simulink model "decimation_filter_o"  (R2019b)
settings: Solver=VariableStepAuto  StartTime=0.0  StopTime=ts*N*(Mpoints/N+200)  RelTol=1e-3
InitFcn:
  | %fs=256*2e4;
  | %osr=512;
  | 
  | osr=1500;
  | fs=6e6;
  | ts=1/fs;
  | 
  | Ncycle=11;
  | Mpoints=2^15;
  | fin=fs*Ncycle/Mpoints;
  | 
  | N=1024;
  | 
  | ref=16/15;
undefined symbols (not defined in the file or in its folder): argo, clock, firhalfband
libraries: SDtoolbox x19, dspfdesign x9, dspmlti4 x9
settings Model: Creator=admin  LastModifiedBy=admin

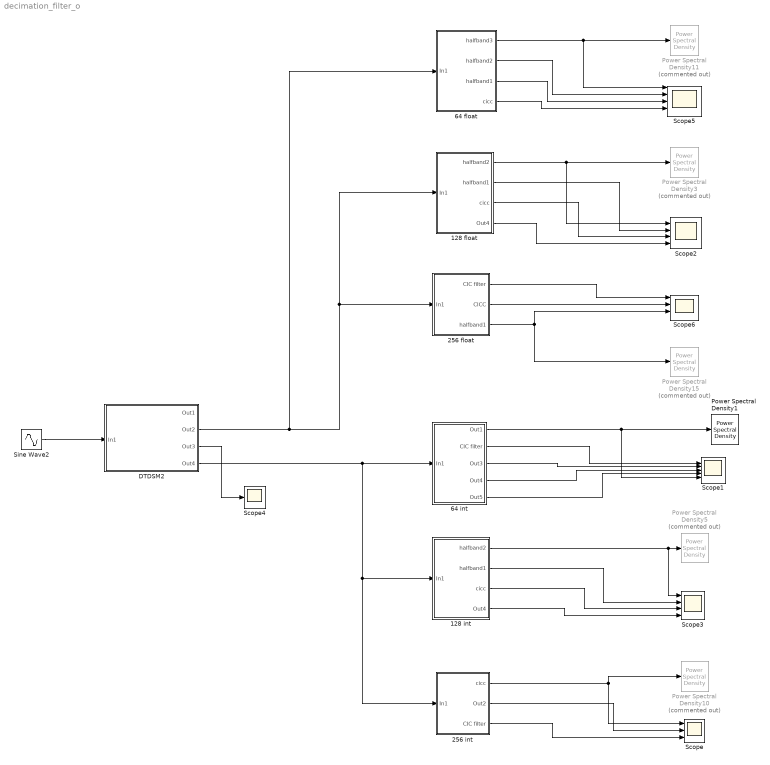
== system decimation_filter_o ==
  "128 float " : Subsystem
  128 int : Subsystem
  256 float : Subsystem
  256 int : Subsystem
  64 float : Subsystem
  64 int : Subsystem
  DTDSM2 : Subsystem
  Power Spectral Density1 : SDtoolbox/Power Spectral Density  SN=7  Fs=fs/1024  fBL=1  fBH=fs/2048  Fin=fin  N=Mpoints/1024  Ntransient=100  VW=on  savename=11  Scale_type=logarithmic
      settings: SourceProductName=SDtoolbox
  Power Spectral Density10 : SDtoolbox/Power Spectral Density  Commented=on  SN=8  Fs=fs/1024  fBL=1  fBH=fs/2048  Fin=fin  N=Mpoints/1024  Ntransient=100  VW=on  savename=11  Scale_type=logarithmic
      settings: SourceProductName=SDtoolbox
  Power Spectral Density11 : SDtoolbox/Power Spectral Density  Commented=on  SN=9  Fs=fs/1024  fBL=1  fBH=fs/2048  Fin=fin  N=Mpoints/1024  Ntransient=100  VW=on  savename=11  Scale_type=logarithmic
      settings: SourceProductName=SDtoolbox
  Power Spectral Density15 : SDtoolbox/Power Spectral Density  Commented=on  SN=10  Fs=fs/1024  fBL=1  fBH=fs/2048  Fin=fin  N=Mpoints/1024  Ntransient=100  VW=on  savename=11  Scale_type=logarithmic
      settings: SourceProductName=SDtoolbox
  Power Spectral Density3 : SDtoolbox/Power Spectral Density  Commented=on  SN=6  Fs=fs/1024  fBL=1  fBH=fs/2048  Fin=fin  N=Mpoints/1024  Ntransient=100  VW=on  savename=11  Scale_type=logarithmic
      settings: SourceProductName=SDtoolbox
  Power Spectral Density5 : SDtoolbox/Power Spectral Density  Commented=on  SN=7  Fs=fs/1024  fBL=1  fBH=fs/2048  Fin=fin  N=Mpoints/1024  Ntransient=100  VW=on  savename=11  Scale_type=logarithmic
      settings: SourceProductName=SDtoolbox
  Scope : Scope  NumInputPorts=3
  Scope1 : Scope  NumInputPorts=5
  Scope2 : Scope  NumInputPorts=4
  Scope3 : Scope  NumInputPorts=4
  Scope4 : Scope
  Scope5 : Scope  NumInputPorts=5
  Scope6 : Scope  NumInputPorts=4
  Sine Wave2 : Sin  Amplitude=0.68  Frequency=fin*2*pi  SampleTime=ts
  wires:
  Sine Wave2/1 -> DTDSM2/1(In1)
  DTDSM2/2(Out2) -> 256 float/1(In1), "128 float "/1(In1), 64 float/1(In1)
  DTDSM2/4(Out4) -> 128 int/1(In1), 256 int/1(In1), 64 int/1(In1)
  "128 float "/1(halfband2) -> Power Spectral Density3/1, Scope2/1
  "128 float "/2(halfband1) -> Scope2/2
  "128 float "/3(cicc) -> Scope2/3
  "128 float "/4(Out4) -> Scope2/4
  128 int/1(halfband2) -> Scope3/1, Power Spectral Density5/1
  128 int/2(halfband1) -> Scope3/2
  128 int/3(cicc) -> Scope3/3
  128 int/4(Out4) -> Scope3/4
  64 float/1(halfband3) -> Power Spectral Density11/1, Scope5/1
  64 float/2(halfband2) -> Scope5/2
  64 float/3(halfband1) -> Scope5/3
  64 float/4(cicc) -> Scope5/4
  256 float/3(halfband1) -> Power Spectral Density15/1, Scope6/3
  256 float/1(CIC filter) -> Scope6/1
  256 float/2(CICC) -> Scope6/2
  256 int/1(cicc) -> Power Spectral Density10/1, Scope/1
  256 int/2(Out2) -> Scope/2
  256 int/3(CIC filter) -> Scope/3
  64 int/2(CIC filter) -> Scope1/1
  64 int/3(Out3) -> Scope1/2
  64 int/4(Out4) -> Scope1/3
  64 int/5(Out5) -> Scope1/4
  DTDSM2/3(Out3) -> Scope4/1
  64 int/1(Out1) -> Power Spectral Density1/1, Scope1/5

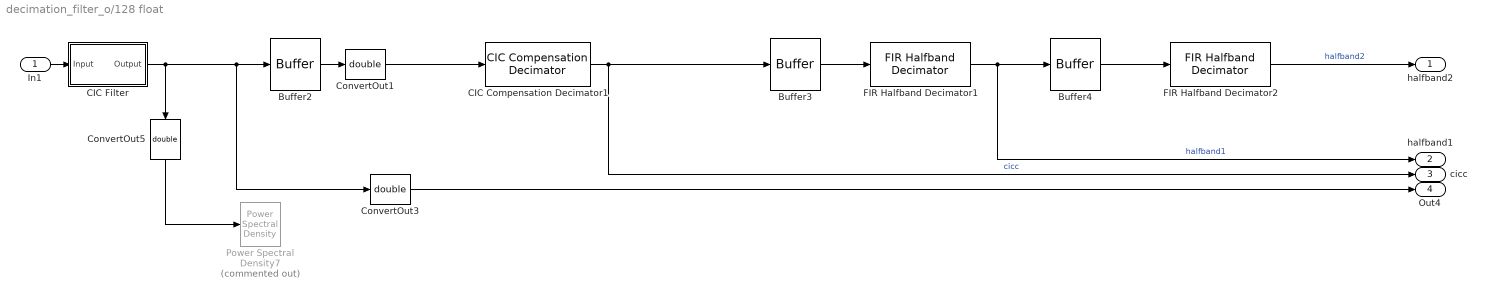
== system decimation_filter_o/128 float  ==
  In1 : Inport
  Buffer2 : Buffer  N=2  OutputFrames=off
  Buffer3 : Buffer  N=2  OutputFrames=off
  Buffer4 : Buffer  N=2  OutputFrames=off
  CIC Compensation Decimator1 : dspfdesign/CIC Compensation Decimator  CICRateChangeFactor=128  CICNumSections=3  CICDifferentialDelay=1  DecimationFactor=2  DesignForMinimumOrder=on  FilterOrder=12  PassbandFrequency=fs/2048  StopbandFrequency=20000  PassbandRipple=0.01  StopbandAttenuation=120  InheritSampleRate=off  SampleRate=23437.5*2  SimulateUsing=Code generation  roundingMode=Floor  coeffsDataTypeStr=fixdt(1,16)
      settings: SourceProductName=DSP System Toolbox  SourceProductBaseCode=DS
  CIC Filter : Subsystem  Tag=FilterWizardSubSystem
      settings: ErrorFcn=dspFilterRealizedInBasicElemsAlgLoopErrFcnCallback
  ConvertOut1 : DataTypeConversion  OutDataTypeStr=double
  ConvertOut3 : DataTypeConversion  OutDataTypeStr=double
  ConvertOut5 : DataTypeConversion  OutDataTypeStr=double
  FIR Halfband Decimator1 : dspfdesign/FIR Halfband Decimator  Specification=Transition width and stopband attenuation  FilterOrder=52  TransitionWidth=6000  StopbandAttenuation=80  Numerator=firhalfband( 'minorder', 0.407, 1e-4 )  FilterBankOutputPort=off  InheritSampleRate=off  SampleRate=fs/256  SimulateUsing=Code generation  roundingMode=Floor  coeffsDataTypeStr=fixdt(1,16)
      settings: SourceProductName=DSP System Toolbox  SourceProductBaseCode=DS
  FIR Halfband Decimator2 : dspfdesign/FIR Halfband Decimator  Specification=Transition width and stopband attenuation  FilterOrder=52  TransitionWidth=3000  StopbandAttenuation=90  Numerator=firhalfband( 'minorder', 0.407, 1e-4 )  FilterBankOutputPort=off  InheritSampleRate=off  SampleRate=fs/512  SimulateUsing=Code generation  roundingMode=Floor  coeffsDataTypeStr=fixdt(1,16)
      settings: SourceProductName=DSP System Toolbox  SourceProductBaseCode=DS
  Power Spectral Density7 : SDtoolbox/Power Spectral Density  Commented=on  SN=5  Fs=fs/128  fBL=1  fBH=fs/2048  Fin=fin  N=Mpoints/128  Ntransient=100  VW=on  savename=11  Scale_type=logarithmic
      settings: SourceProductName=SDtoolbox
  halfband2 : Outport
  halfband1 : Outport  Port=2
  cicc : Outport  Port=3
  Out4 : Outport  Port=4
  wires:
  ConvertOut1/1 -> CIC Compensation Decimator1/1
  Buffer3/1 -> FIR Halfband Decimator1/1
  CIC Filter/1(Output) -> ConvertOut5/1, Buffer2/1, ConvertOut3/1
  FIR Halfband Decimator2/1 -> halfband2/1  "halfband2"
  FIR Halfband Decimator1/1 -> halfband1/1, Buffer4/1  "halfband1"
  ConvertOut5/1 -> Power Spectral Density7/1
  Buffer2/1 -> ConvertOut1/1
  Buffer4/1 -> FIR Halfband Decimator2/1
  CIC Compensation Decimator1/1 -> cicc/1, Buffer3/1  "cicc"
  ConvertOut3/1 -> Out4/1
  In1/1 -> CIC Filter/1(Input)

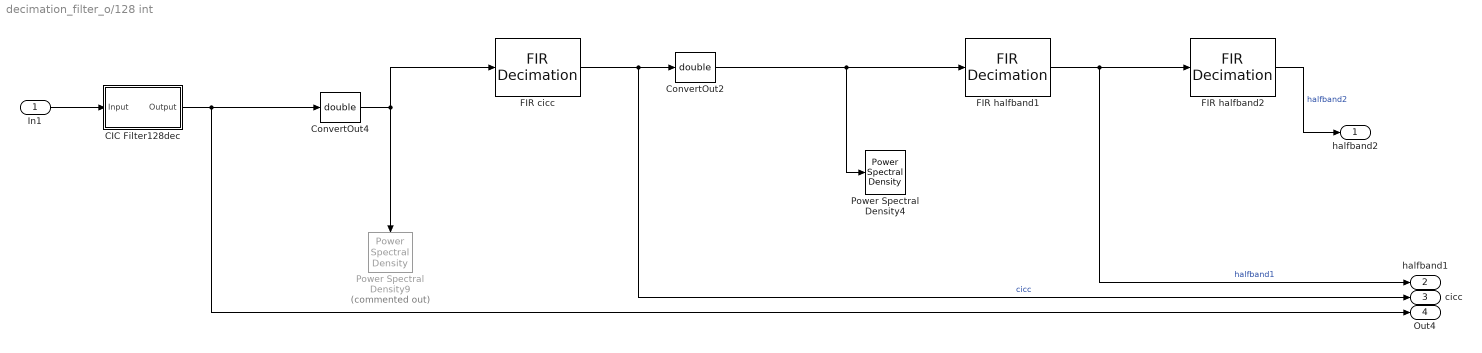
== system decimation_filter_o/128 int ==
  In1 : Inport
  CIC Filter128dec : Subsystem  Tag=FilterWizardSubSystem
      settings: ErrorFcn=dspFilterRealizedInBasicElemsAlgLoopErrFcnCallback
  ConvertOut2 : DataTypeConversion  OutDataTypeStr=double
  ConvertOut4 : DataTypeConversion  OutDataTypeStr=double
  FIR cicc : dspmlti4/FIR Decimation  FilterSource=Dialog parameters  h=coff_ciccom_round_128m  D=2  filtStruct=Direct form  FilterObject=FDECIM  framing=Allow multirate processing  inputOffset=0  outputBufInitCond=0  roundingMode=Ceiling  overflowMode=off  firstCoeffDataTypeStr=Inherit: Same word length as input  firstCoeffMin=[]  firstCoeffMax=[]  firstCoeffLastDataTypeStr=Inherit: Same word length as input  outputMin=[]  outputMax=[]
  FIR halfband1 : dspmlti4/FIR Decimation  FilterSource=Dialog parameters  h=half1co_r_128m  D=2  filtStruct=Direct form  FilterObject=FDECIM  framing=Allow multirate processing  inputOffset=0  outputBufInitCond=0  roundingMode=Ceiling  overflowMode=off  firstCoeffDataTypeStr=Inherit: Same word length as input  firstCoeffMin=[]  firstCoeffMax=[]  firstCoeffLastDataTypeStr=Inherit: Same word length as input  outputMin=[]  outputMax=[]
  FIR halfband2 : dspmlti4/FIR Decimation  FilterSource=Dialog parameters  h=half2co_r_128m  D=2  filtStruct=Direct form  FilterObject=FDECIM  framing=Allow multirate processing  inputOffset=0  outputBufInitCond=0  roundingMode=Ceiling  overflowMode=off  firstCoeffDataTypeStr=Inherit: Same word length as input  firstCoeffMin=[]  firstCoeffMax=[]  firstCoeffLastDataTypeStr=Inherit: Same word length as input  outputMin=[]  outputMax=[]
  Power Spectral Density4 : SDtoolbox/Power Spectral Density  SN=5  Fs=fs/256  fBL=1  fBH=fs/2048  Fin=fin  N=Mpoints/256  Ntransient=100  VW=on  savename=11  Scale_type=logarithmic
      settings: SourceProductName=SDtoolbox
  Power Spectral Density9 : SDtoolbox/Power Spectral Density  Commented=on  SN=5  Fs=fs/128  fBL=1  fBH=fs/2048  Fin=fin  N=Mpoints/128  Ntransient=100  VW=on  savename=11  Scale_type=logarithmic
      settings: SourceProductName=SDtoolbox
  halfband2 : Outport
  halfband1 : Outport  Port=2
  cicc : Outport  Port=3
  Out4 : Outport  Port=4
  wires:
  In1/1 -> CIC Filter128dec/1(Input)
  FIR halfband1/1 -> halfband1/1, FIR halfband2/1  "halfband1"
  FIR cicc/1 -> cicc/1, ConvertOut2/1  "cicc"
  ConvertOut4/1 -> Power Spectral Density9/1, FIR cicc/1
  FIR halfband2/1 -> halfband2/1  "halfband2"
  CIC Filter128dec/1(Output) -> Out4/1, ConvertOut4/1
  ConvertOut2/1 -> Power Spectral Density4/1, FIR halfband1/1

== system decimation_filter_o/256 float ==
  In1 : Inport
  Buffer10 : Buffer  N=2  OutputFrames=off
  Buffer9 : Buffer  N=2  OutputFrames=off
  CIC Compensation Decimator3 : dspfdesign/CIC Compensation Decimator  CICRateChangeFactor=256  CICNumSections=3  CICDifferentialDelay=1  DecimationFactor=2  DesignForMinimumOrder=on  FilterOrder=12  PassbandFrequency=fs/2048  StopbandFrequency=10000  PassbandRipple=0.01  StopbandAttenuation=120  InheritSampleRate=off  SampleRate=23437.5  SimulateUsing=Code generation  roundingMode=Floor  coeffsDataTypeStr=fixdt(1,16)
      settings: SourceProductName=DSP System Toolbox  SourceProductBaseCode=DS
  ConvertOut9 : DataTypeConversion  OutDataTypeStr=double
  FIR Halfband Decimator6 : dspfdesign/FIR Halfband Decimator  Specification=Transition width and stopband attenuation  FilterOrder=52  TransitionWidth=4000  StopbandAttenuation=90  Numerator=firhalfband( 'minorder', 0.407, 1e-4 )  FilterBankOutputPort=off  InheritSampleRate=off  SampleRate=fs/512  SimulateUsing=Code generation  roundingMode=Floor  coeffsDataTypeStr=fixdt(1,16)
      settings: SourceProductName=DSP System Toolbox  SourceProductBaseCode=DS
  Filter1 : Subsystem  Tag=FilterWizardSubSystem
      settings: ErrorFcn=dspFilterRealizedInBasicElemsAlgLoopErrFcnCallback
  Power Spectral Density12 : SDtoolbox/Power Spectral Density  Commented=on  SN=3  Fs=fs/256  fBL=1  fBH=fs/2048  Fin=fin  N=Mpoints/256  Ntransient=10  VW=on  savename=11  Scale_type=logarithmic
      settings: SourceProductName=SDtoolbox
  Power Spectral Density13 : SDtoolbox/Power Spectral Density  Commented=on  SN=4  Fs=fs/512  fBL=1  fBH=fs/2048  Fin=fin  N=Mpoints/512  Ntransient=10  VW=on  savename=11  Scale_type=logarithmic
      settings: SourceProductName=SDtoolbox
  CIC filter : Outport
  CICC : Outport  Port=2
  halfband1 : Outport  Port=3
  wires:
  ConvertOut9/1 -> Power Spectral Density12/1, CIC Compensation Decimator3/1
  CIC Compensation Decimator3/1 -> CICC/1, Buffer10/1, Power Spectral Density13/1  "CICC"
  Filter1/1(Output) -> CIC filter/1, Buffer9/1  "CIC filter"
  Buffer9/1 -> ConvertOut9/1
  Buffer10/1 -> FIR Halfband Decimator6/1
  In1/1 -> Filter1/1(Input)
  FIR Halfband Decimator6/1 -> halfband1/1  "halfband1"

== system decimation_filter_o/256 int ==
  In1 : Inport
  CIC Filter256dec : Subsystem  Tag=FilterWizardSubSystem
      settings: ErrorFcn=dspFilterRealizedInBasicElemsAlgLoopErrFcnCallback
  ConvertOut6 : DataTypeConversion  OutDataTypeStr=double
  FIR cicc1 : dspmlti4/FIR Decimation  FilterSource=Dialog parameters  h=coff_ciccom_round_256m  D=2  filtStruct=Direct form  FilterObject=FDECIM  framing=Allow multirate processing  inputOffset=0  outputBufInitCond=0  roundingMode=Ceiling  overflowMode=off  firstCoeffDataTypeStr=Inherit: Same word length as input  firstCoeffMin=[]  firstCoeffMax=[]  firstCoeffLastDataTypeStr=Inherit: Same word length as input  outputMin=[]  outputMax=[]
  FIR halfband : dspmlti4/FIR Decimation  FilterSource=Dialog parameters  h=half1co_r_256m  D=2  filtStruct=Direct form  FilterObject=FDECIM  framing=Allow multirate processing  inputOffset=0  outputBufInitCond=0  roundingMode=Ceiling  overflowMode=off  firstCoeffDataTypeStr=Inherit: Same word length as input  firstCoeffMin=[]  firstCoeffMax=[]  firstCoeffLastDataTypeStr=Inherit: Same word length as input  outputMin=[]  outputMax=[]
  Power Spectral Density6 : SDtoolbox/Power Spectral Density  Commented=on  SN=5  Fs=fs/256  fBL=1  fBH=fs/2048  Fin=fin  N=Mpoints/256  Ntransient=100  VW=on  savename=11  Scale_type=logarithmic
      settings: SourceProductName=SDtoolbox
  cicc : Outport
  Out2 : Outport  Port=2
  CIC filter : Outport  Port=3
  wires:
  ConvertOut6/1 -> Power Spectral Density6/1, FIR cicc1/1
  FIR cicc1/1 -> Out2/1, FIR halfband/1
  In1/1 -> CIC Filter256dec/1(Input)
  CIC Filter256dec/1(Output) -> CIC filter/1, ConvertOut6/1  "CIC filter"
  FIR halfband/1 -> cicc/1  "cicc"

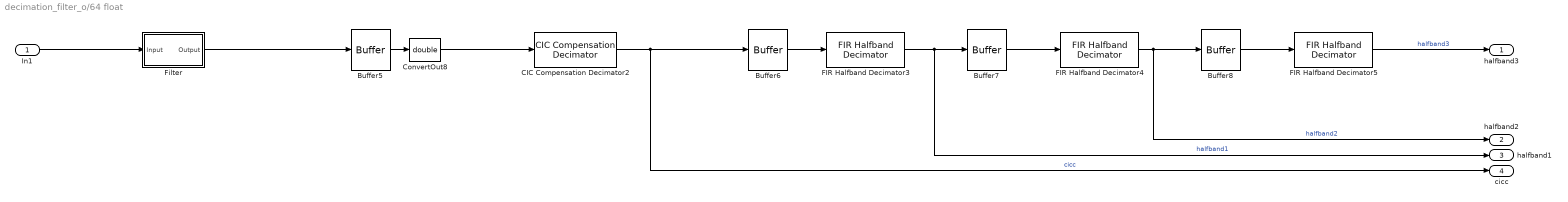
== system decimation_filter_o/64 float ==
  In1 : Inport
  Buffer{5..8} (4 alike) : Buffer  N=2  OutputFrames=off
  CIC Compensation Decimator2 : dspfdesign/CIC Compensation Decimator  CICRateChangeFactor=64  CICNumSections=3  CICDifferentialDelay=1  DecimationFactor=2  DesignForMinimumOrder=on  FilterOrder=12  PassbandFrequency=fs/2048  StopbandFrequency=40000  PassbandRipple=0.01  StopbandAttenuation=120  InheritSampleRate=off  SampleRate=23437.5*4  SimulateUsing=Code generation  roundingMode=Floor  coeffsDataTypeStr=fixdt(1,16)
      settings: SourceProductName=DSP System Toolbox  SourceProductBaseCode=DS
  ConvertOut8 : DataTypeConversion  OutDataTypeStr=double
  FIR Halfband Decimator3 : dspfdesign/FIR Halfband Decimator  Specification=Transition width and stopband attenuation  FilterOrder=52  TransitionWidth=16000  StopbandAttenuation=80  Numerator=firhalfband( 'minorder', 0.407, 1e-4 )  FilterBankOutputPort=off  InheritSampleRate=off  SampleRate=fs/128  SimulateUsing=Code generation  roundingMode=Floor  coeffsDataTypeStr=fixdt(1,16)
      settings: SourceProductName=DSP System Toolbox  SourceProductBaseCode=DS
  FIR Halfband Decimator4 : dspfdesign/FIR Halfband Decimator  Specification=Transition width and stopband attenuation  FilterOrder=52  TransitionWidth=10000  StopbandAttenuation=90  Numerator=firhalfband( 'minorder', 0.407, 1e-4 )  FilterBankOutputPort=off  InheritSampleRate=off  SampleRate=fs/256  SimulateUsing=Code generation  roundingMode=Floor  coeffsDataTypeStr=fixdt(1,16)
      settings: SourceProductName=DSP System Toolbox  SourceProductBaseCode=DS
  FIR Halfband Decimator5 : dspfdesign/FIR Halfband Decimator  Specification=Transition width and stopband attenuation  FilterOrder=52  TransitionWidth=3500  StopbandAttenuation=100  Numerator=firhalfband( 'minorder', 0.407, 1e-4 )  FilterBankOutputPort=off  InheritSampleRate=off  SampleRate=fs/512  SimulateUsing=Code generation  roundingMode=Floor  coeffsDataTypeStr=fixdt(1,16)
      settings: SourceProductName=DSP System Toolbox  SourceProductBaseCode=DS
  Filter : Subsystem  Tag=FilterWizardSubSystem
      settings: ErrorFcn=dspFilterRealizedInBasicElemsAlgLoopErrFcnCallback
  halfband3 : Outport
  halfband2 : Outport  Port=2
  halfband1 : Outport  Port=3
  cicc : Outport  Port=4
  wires:
  Buffer8/1 -> FIR Halfband Decimator5/1
  Buffer7/1 -> FIR Halfband Decimator4/1
  FIR Halfband Decimator4/1 -> halfband2/1, Buffer8/1  "halfband2"
  Filter/1(Output) -> Buffer5/1
  CIC Compensation Decimator2/1 -> cicc/1, Buffer6/1  "cicc"
  FIR Halfband Decimator3/1 -> halfband1/1, Buffer7/1  "halfband1"
  Buffer6/1 -> FIR Halfband Decimator3/1
  Buffer5/1 -> ConvertOut8/1
  ConvertOut8/1 -> CIC Compensation Decimator2/1
  FIR Halfband Decimator5/1 -> halfband3/1  "halfband3"
  In1/1 -> Filter/1(Input)

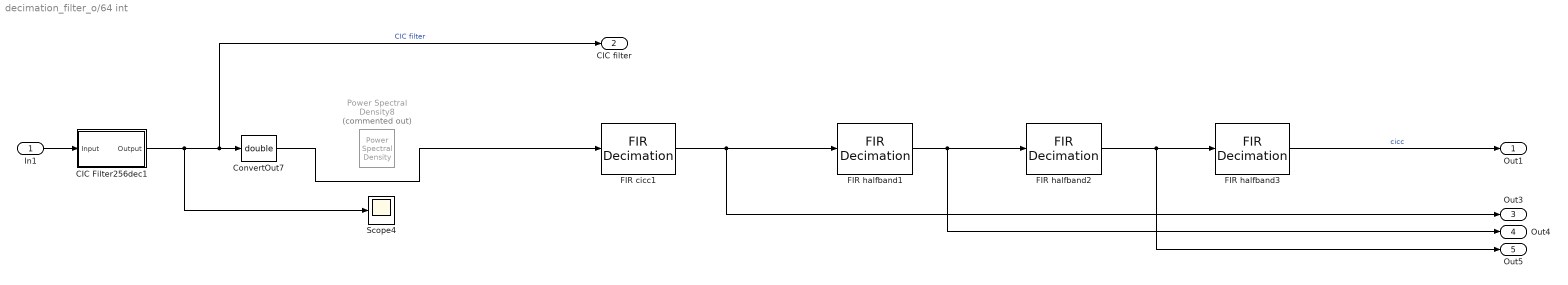
== system decimation_filter_o/64 int ==
  In1 : Inport
  CIC Filter256dec1 : Subsystem  Tag=FilterWizardSubSystem
      settings: ErrorFcn=dspFilterRealizedInBasicElemsAlgLoopErrFcnCallback
  ConvertOut7 : DataTypeConversion  OutDataTypeStr=double
  FIR cicc1 : dspmlti4/FIR Decimation  FilterSource=Dialog parameters  h=coff_ciccom_round_64m  D=2  filtStruct=Direct form  FilterObject=FDECIM  framing=Allow multirate processing  inputOffset=0  outputBufInitCond=0  roundingMode=Ceiling  overflowMode=off  firstCoeffDataTypeStr=Inherit: Same word length as input  firstCoeffMin=[]  firstCoeffMax=[]  firstCoeffLastDataTypeStr=Inherit: Same word length as input  outputMin=[]  outputMax=[]
  FIR halfband1 : dspmlti4/FIR Decimation  FilterSource=Dialog parameters  h=half1co_r_64m  D=2  filtStruct=Direct form  FilterObject=FDECIM  framing=Allow multirate processing  inputOffset=0  outputBufInitCond=0  roundingMode=Ceiling  overflowMode=off  firstCoeffDataTypeStr=Inherit: Same word length as input  firstCoeffMin=[]  firstCoeffMax=[]  firstCoeffLastDataTypeStr=Inherit: Same word length as input  outputMin=[]  outputMax=[]
  FIR halfband2 : dspmlti4/FIR Decimation  FilterSource=Dialog parameters  h=half2co_r_64m  D=2  filtStruct=Direct form  FilterObject=FDECIM  framing=Allow multirate processing  inputOffset=0  outputBufInitCond=0  roundingMode=Ceiling  overflowMode=off  firstCoeffDataTypeStr=Inherit: Same word length as input  firstCoeffMin=[]  firstCoeffMax=[]  firstCoeffLastDataTypeStr=Inherit: Same word length as input  outputMin=[]  outputMax=[]
  FIR halfband3 : dspmlti4/FIR Decimation  FilterSource=Dialog parameters  h=half3co_r_64m  D=2  filtStruct=Direct form  FilterObject=FDECIM  framing=Allow multirate processing  inputOffset=0  outputBufInitCond=0  roundingMode=Ceiling  overflowMode=off  firstCoeffDataTypeStr=Inherit: Same word length as input  firstCoeffMin=[]  firstCoeffMax=[]  firstCoeffLastDataTypeStr=Inherit: Same word length as input  outputMin=[]  outputMax=[]
  Power Spectral Density8 : SDtoolbox/Power Spectral Density  Commented=on  SN=5  Fs=fs/64  fBL=1  fBH=fs/2048  Fin=fin  N=Mpoints/64  Ntransient=100  VW=on  savename=11  Scale_type=logarithmic
      settings: SourceProductName=SDtoolbox
  Scope4 : Scope
  Out1 : Outport
  CIC filter : Outport  Port=2
  Out3 : Outport  Port=3
  Out4 : Outport  Port=4
  Out5 : Outport  Port=5
  wires:
  FIR cicc1/1 -> Out3/1, FIR halfband1/1
  FIR halfband3/1 -> Out1/1  "cicc"
  FIR halfband2/1 -> Out5/1, FIR halfband3/1
  CIC Filter256dec1/1(Output) -> Scope4/1, CIC filter/1, ConvertOut7/1  "CIC filter"
  FIR halfband1/1 -> Out4/1, FIR halfband2/1
  In1/1 -> CIC Filter256dec1/1(Input)
  ConvertOut7/1 -> FIR cicc1/1

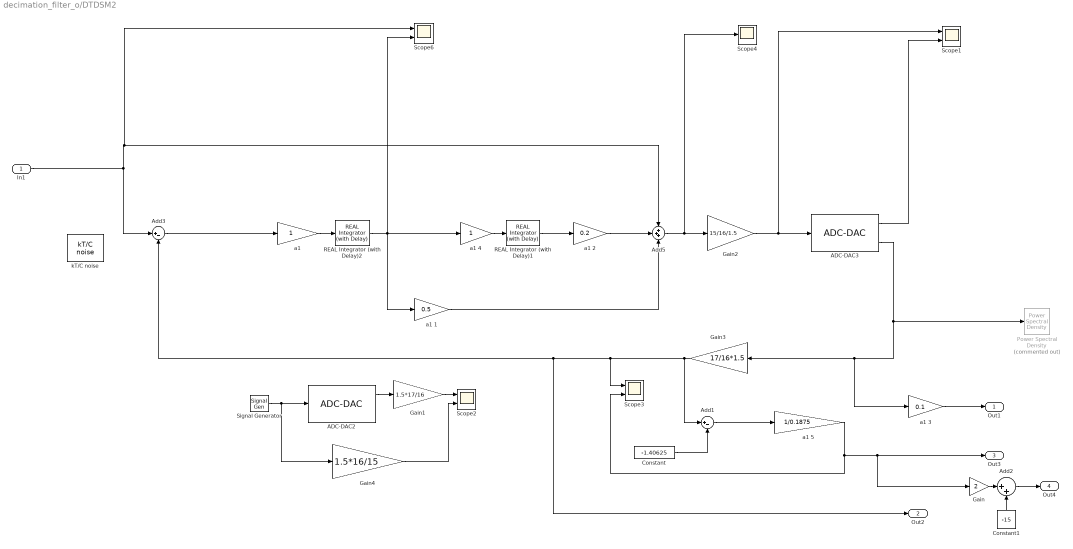
== system decimation_filter_o/DTDSM2 ==
  In1 : Inport
  ADC-DAC2 : SDtoolbox/ADC-DAC  k=17  MM=off  match=0  CST=0  VVG=off  argo=argo(:,3)  LF=on  NF=retA.log
      settings: SourceProductName=SDtoolbox
  ADC-DAC3 : SDtoolbox/ADC-DAC  k=17  MM=off  match=0  CST=0  VVG=off  argo=argo(:,3)  LF=on  NF=retA.log
      settings: SourceProductName=SDtoolbox
  Add1 : Sum  Inputs=|+-
  Add2 : Sum  Inputs=|++
  Add3 : Sum  Inputs=|+-
  Add5 : Sum  Inputs=+++
  Constant : Constant  Value=-1.40625
  Constant1 : Constant  Value=-15
  Gain : Gain  Gain=2
  Gain1 : Gain  Gain=1.5*17/16
  Gain2 : Gain  Gain=15/16/1.5
  Gain3 : Gain  Gain=17/16*1.5
  Gain4 : Gain  Gain=1.5*16/15
  Power Spectral Density : SDtoolbox/Power Spectral Density  Commented=on  SN=3  Fs=fs  fBL=1  fBH=fs/2048  Fin=fin  N=Mpoints  Ntransient=10  VW=on  savename=11  Scale_type=logarithmic
      settings: SourceProductName=SDtoolbox
  REAL Integrator (with Delay)1 : SDtoolbox/REAL Integrator (with Delay)  Ts=ts  alfa=(1e4-1)/1e4  Amax=1  sr=1e7  GBW=1e8
      settings: SourceProductName=SDtoolbox
  REAL Integrator (with Delay)2 : SDtoolbox/REAL Integrator (with Delay)  Ts=ts  alfa=(1e4-1)/1e4  Amax=3.3  sr=1E8  GBW=1E7
      settings: SourceProductName=SDtoolbox
  Scope{1..3,6} (4 alike) : Scope  NumInputPorts=2
  Scope4 : Scope
  Signal Generator : SignalGenerator  WaveForm=sawtooth  Frequency=5000  Units=rad/sec
  "a1 " : Gain
  a1 1 : Gain  Gain=0.5
  a1 2 : Gain  Gain=0.2
  a1 3 : Gain  Gain=0.1
  a1 4 : Gain
  a1 5 : Gain  Gain=1/0.1875
  kT/C noise : SDtoolbox/kT//C noise  Ts=ts  C=16e-12  Temp=300  k=1.38e-23  seed=floor(sum(clock))
      settings: SourceProductName=SDtoolbox
  Out1 : Outport
  Out2 : Outport  Port=2
  Out3 : Outport  Port=3
  Out4 : Outport  Port=4
  wires:
  Gain2/1 -> ADC-DAC3/1, Scope1/1
  Add3/1 -> "a1 "/1
  REAL Integrator (with Delay)1/1 -> a1 2/1
  Gain1/1 -> Scope2/1
  a1 2/1 -> Add5/2
  a1 4/1 -> REAL Integrator (with Delay)1/1
  In1/1 -> Add3/1, Add5/1, Scope6/1
  "a1 "/1 -> REAL Integrator (with Delay)2/1
  Add5/1 -> Scope4/1, Gain2/1
  Signal Generator/1 -> Gain4/1, ADC-DAC2/1
  ADC-DAC3/1 -> Scope1/2
  REAL Integrator (with Delay)2/1 -> a1 4/1, Scope6/2, a1 1/1
  ADC-DAC2/1 -> Gain1/1
  a1 1/1 -> Add5/3
  Gain4/1 -> Scope2/2
  ADC-DAC3/2 -> Power Spectral Density/1, a1 3/1, Gain3/1
  a1 3/1 -> Out1/1
  Gain3/1 -> Add1/1, Scope3/1, Out2/1, Add3/2
  Constant/1 -> Add1/2
  Add1/1 -> a1 5/1
  a1 5/1 -> Gain/1, Out3/1, Scope3/2
  Constant1/1 -> Add2/2
  Gain/1 -> Add2/1
  Add2/1 -> Out4/1

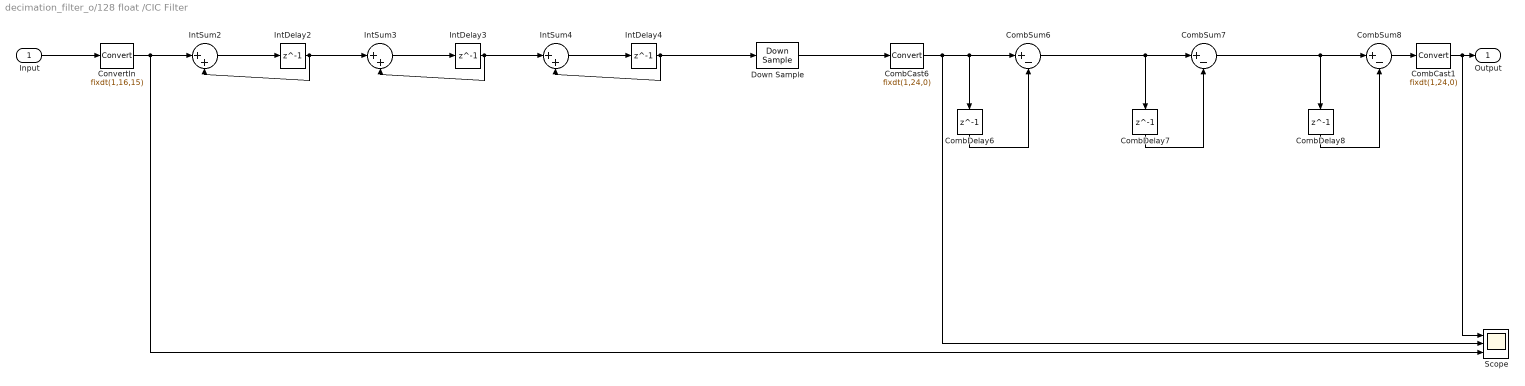
== system decimation_filter_o/128 float /CIC Filter ==
  Input : Inport
  CombCast1 : DataTypeConversion  OutDataTypeStr=fixdt(1,24,0)
  CombCast6 : DataTypeConversion  OutDataTypeStr=fixdt(1,24,0)
  CombDelay6 : Delay  DelayLength=1  InitialCondition=0
  CombDelay7 : Delay  DelayLength=1  InitialCondition=0
  CombDelay8 : Delay  DelayLength=1  InitialCondition=0
  CombSum6 : Sum  Inputs=|+-  AccumDataTypeStr=fixdt(1,37,15)  OutDataTypeStr=fixdt(1,37,15)
  CombSum7 : Sum  Inputs=|+-  AccumDataTypeStr=fixdt(1,37,15)  OutDataTypeStr=fixdt(1,37,15)
  CombSum8 : Sum  Inputs=|+-  AccumDataTypeStr=fixdt(1,37,15)  OutDataTypeStr=fixdt(1,37,15)
  ConvertIn : DataTypeConversion  OutDataTypeStr=fixdt(1,16,15)  RndMeth=Nearest  SaturateOnIntegerOverflow=on
  Down Sample : DownSample  N=128  RateOptions=Allow multirate processing
  IntDelay2 : Delay  DelayLength=1  InitialCondition=0
  IntDelay3 : Delay  DelayLength=1  InitialCondition=0
  IntDelay4 : Delay  DelayLength=1  InitialCondition=0
  IntSum2 : Sum  Inputs=|++  AccumDataTypeStr=fixdt(1,37,15)  OutDataTypeStr=fixdt(1,37,15)
  IntSum3 : Sum  Inputs=|++  AccumDataTypeStr=fixdt(1,37,15)  OutDataTypeStr=fixdt(1,37,15)
  IntSum4 : Sum  Inputs=|++  AccumDataTypeStr=fixdt(1,37,15)  OutDataTypeStr=fixdt(1,37,15)
  Scope : Scope  NumInputPorts=3
  Output : Outport
  wires:
  Input/1 -> ConvertIn/1
  ConvertIn/1 -> Scope/3, IntSum2/1
  IntSum2/1 -> IntDelay2/1
  IntDelay2/1 -> IntSum2/2, IntSum3/1
  IntSum3/1 -> IntDelay3/1
  IntDelay3/1 -> IntSum3/2, IntSum4/1
  IntSum4/1 -> IntDelay4/1
  IntDelay4/1 -> IntSum4/2, Down Sample/1
  Down Sample/1 -> CombCast6/1
  CombSum6/1 -> CombSum7/1, CombDelay7/1
  CombDelay6/1 -> CombSum6/2
  CombCast6/1 -> Scope/2, CombSum6/1, CombDelay6/1
  CombSum7/1 -> CombSum8/1, CombDelay8/1
  CombDelay7/1 -> CombSum7/2
  CombSum8/1 -> CombCast1/1
  CombDelay8/1 -> CombSum8/2
  CombCast1/1 -> Scope/1, Output/1

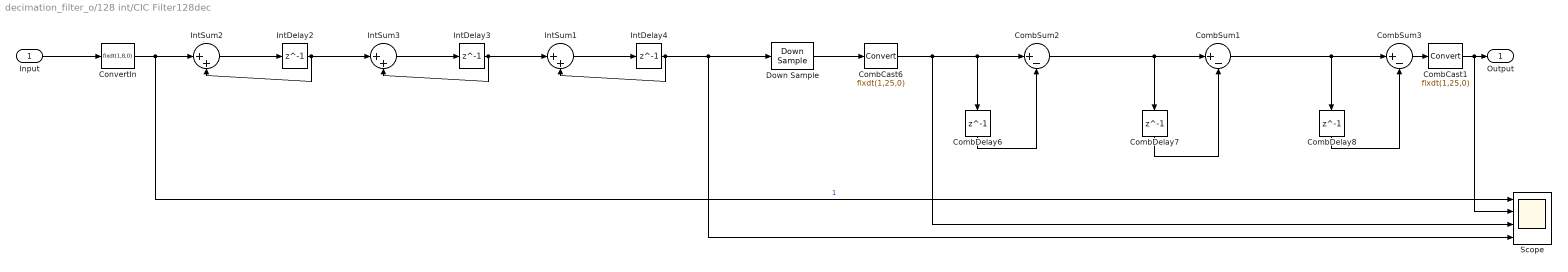
== system decimation_filter_o/128 int/CIC Filter128dec ==
  Input : Inport
  CombCast1 : DataTypeConversion  OutDataTypeStr=fixdt(1,25,0)
  CombCast6 : DataTypeConversion  OutDataTypeStr=fixdt(1,25,0)
  CombDelay6 : Delay  DelayLength=1  InitialCondition=0
  CombDelay7 : Delay  DelayLength=1  InitialCondition=0
  CombDelay8 : Delay  DelayLength=1  InitialCondition=0
  CombSum1 : Sum  Inputs=|+-  AccumDataTypeStr=fixdt(1,25,0)  OutDataTypeStr=fixdt(1,26,0)
  CombSum2 : Sum  Inputs=|+-  AccumDataTypeStr=fixdt(1,25,0)  OutDataTypeStr=fixdt(1,26,0)
  CombSum3 : Sum  Inputs=|+-  AccumDataTypeStr=fixdt(1,25,0)  OutDataTypeStr=fixdt(1,26,0)
  ConvertIn : DataTypeConversion  OutDataTypeStr=fixdt(1,8,0)  RndMeth=Nearest
  Down Sample : DownSample  N=128  RateOptions=Allow multirate processing
  IntDelay2 : Delay  DelayLength=1  InitialCondition=0
  IntDelay3 : Delay  DelayLength=1  InitialCondition=0
  IntDelay4 : Delay  DelayLength=1  InitialCondition=0
  IntSum1 : Sum  Inputs=|++  AccumDataTypeStr=fixdt(1,26,0)  OutDataTypeStr=fixdt(1,26,0)
  IntSum2 : Sum  Inputs=|++  AccumDataTypeStr=fixdt(1,24,0)  OutDataTypeStr=fixdt(1,26,0)
  IntSum3 : Sum  Inputs=|++  AccumDataTypeStr=fixdt(1,26,0)  OutDataTypeStr=fixdt(1,26,0)
  Scope : Scope  NumInputPorts=4
  Output : Outport
  wires:
  ConvertIn/1 -> Scope/1, IntSum2/1  "1"
  IntSum2/1 -> IntDelay2/1
  IntDelay2/1 -> IntSum3/1, IntSum2/2
  IntSum3/1 -> IntDelay3/1
  IntDelay3/1 -> IntSum1/1, IntSum3/2
  IntSum1/1 -> IntDelay4/1
  Down Sample/1 -> CombCast6/1
  CombSum2/1 -> CombSum1/1, CombDelay7/1
  CombDelay6/1 -> CombSum2/2
  CombCast6/1 -> Scope/3, CombSum2/1, CombDelay6/1
  CombSum1/1 -> CombSum3/1, CombDelay8/1
  CombDelay7/1 -> CombSum1/2
  CombSum3/1 -> CombCast1/1
  CombDelay8/1 -> CombSum3/2
  CombCast1/1 -> Scope/2, Output/1
  Input/1 -> ConvertIn/1
  IntDelay4/1 -> IntSum1/2, Scope/4, Down Sample/1

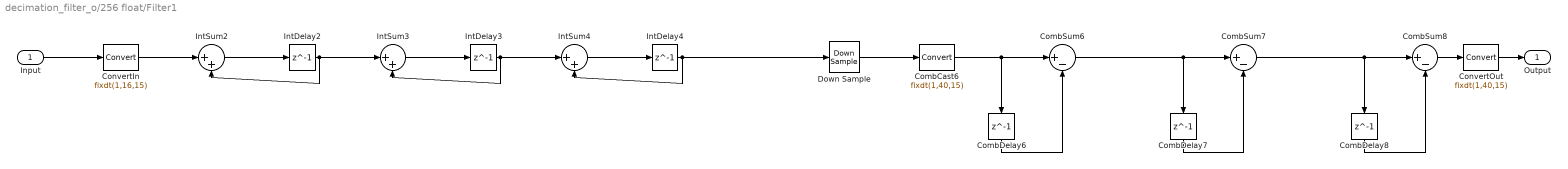
== system decimation_filter_o/256 float/Filter1 ==
  Input : Inport
  CombCast6 : DataTypeConversion  OutDataTypeStr=fixdt(1,40,15)
  CombDelay6 : Delay  DelayLength=1  InitialCondition=0
  CombDelay7 : Delay  DelayLength=1  InitialCondition=0
  CombDelay8 : Delay  DelayLength=1  InitialCondition=0
  CombSum6 : Sum  Inputs=|+-  AccumDataTypeStr=fixdt(1,40,15)  OutDataTypeStr=fixdt(1,40,15)
  CombSum7 : Sum  Inputs=|+-  AccumDataTypeStr=fixdt(1,40,15)  OutDataTypeStr=fixdt(1,40,15)
  CombSum8 : Sum  Inputs=|+-  AccumDataTypeStr=fixdt(1,40,15)  OutDataTypeStr=fixdt(1,40,15)
  ConvertIn : DataTypeConversion  OutDataTypeStr=fixdt(1,16,15)  RndMeth=Nearest  SaturateOnIntegerOverflow=on
  ConvertOut : DataTypeConversion  OutDataTypeStr=fixdt(1,40,15)
  Down Sample : DownSample  N=256  RateOptions=Allow multirate processing
  IntDelay2 : Delay  DelayLength=1  InitialCondition=0
  IntDelay3 : Delay  DelayLength=1  InitialCondition=0
  IntDelay4 : Delay  DelayLength=1  InitialCondition=0
  IntSum2 : Sum  Inputs=|++  AccumDataTypeStr=fixdt(1,40,15)  OutDataTypeStr=fixdt(1,40,15)
  IntSum3 : Sum  Inputs=|++  AccumDataTypeStr=fixdt(1,40,15)  OutDataTypeStr=fixdt(1,40,15)
  IntSum4 : Sum  Inputs=|++  AccumDataTypeStr=fixdt(1,40,15)  OutDataTypeStr=fixdt(1,40,15)
  Output : Outport
  wires:
  Input/1 -> ConvertIn/1
  ConvertIn/1 -> IntSum2/1
  IntSum2/1 -> IntDelay2/1
  IntDelay2/1 -> IntSum2/2, IntSum3/1
  IntSum3/1 -> IntDelay3/1
  IntDelay3/1 -> IntSum3/2, IntSum4/1
  IntSum4/1 -> IntDelay4/1
  IntDelay4/1 -> IntSum4/2, Down Sample/1
  Down Sample/1 -> CombCast6/1
  CombSum6/1 -> CombSum7/1, CombDelay7/1
  CombDelay6/1 -> CombSum6/2
  CombCast6/1 -> CombSum6/1, CombDelay6/1
  CombSum7/1 -> CombSum8/1, CombDelay8/1
  CombDelay7/1 -> CombSum7/2
  CombSum8/1 -> ConvertOut/1
  CombDelay8/1 -> CombSum8/2
  ConvertOut/1 -> Output/1

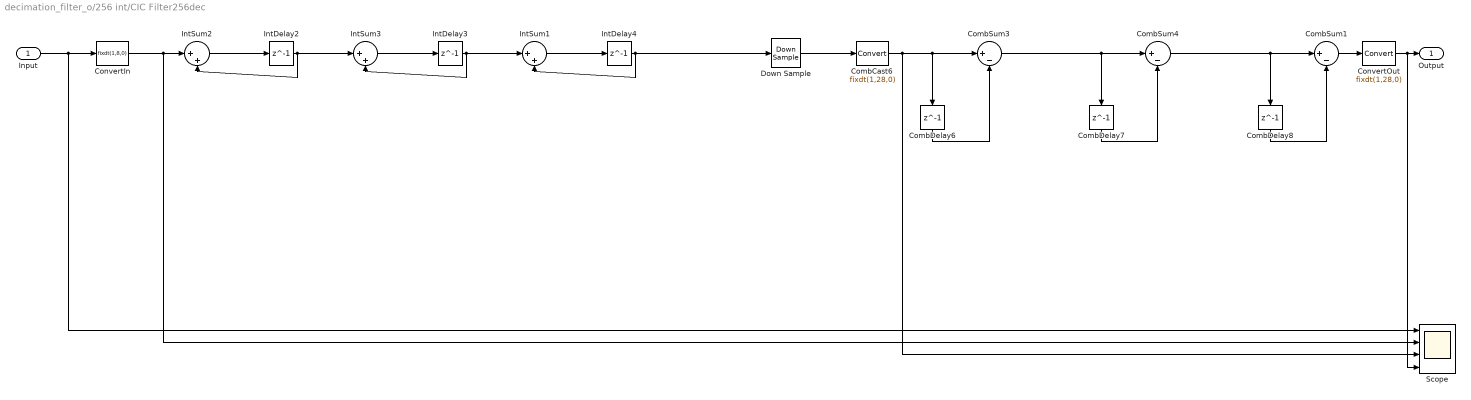
== system decimation_filter_o/256 int/CIC Filter256dec ==
  Input : Inport
  CombCast6 : DataTypeConversion  OutDataTypeStr=fixdt(1,28,0)
  CombDelay6 : Delay  DelayLength=1  InitialCondition=0
  CombDelay7 : Delay  DelayLength=1  InitialCondition=0
  CombDelay8 : Delay  DelayLength=1  InitialCondition=0
  CombSum1 : Sum  Inputs=|+-  AccumDataTypeStr=fixdt(1,28,0)  OutDataTypeStr=fixdt(1,28,0)
  CombSum3 : Sum  Inputs=|+-  AccumDataTypeStr=fixdt(1,28,0)  OutDataTypeStr=fixdt(1,28,0)
  CombSum4 : Sum  Inputs=|+-  AccumDataTypeStr=fixdt(1,28,0)  OutDataTypeStr=fixdt(1,28,0)
  ConvertIn : DataTypeConversion  OutDataTypeStr=fixdt(1,8,0)  RndMeth=Nearest  SaturateOnIntegerOverflow=on
  ConvertOut : DataTypeConversion  OutDataTypeStr=fixdt(1,28,0)
  Down Sample : DownSample  N=256  RateOptions=Allow multirate processing
  IntDelay2 : Delay  DelayLength=1  InitialCondition=0
  IntDelay3 : Delay  DelayLength=1  InitialCondition=0
  IntDelay4 : Delay  DelayLength=1  InitialCondition=0
  IntSum1 : Sum  Inputs=|++  AccumDataTypeStr=fixdt(1,30,0)  OutDataTypeStr=fixdt(1,30,0)
  IntSum2 : Sum  Inputs=|++  AccumDataTypeStr=fixdt(1,30,0)  OutDataTypeStr=fixdt(1,30,0)
  IntSum3 : Sum  Inputs=|++  AccumDataTypeStr=fixdt(1,30,0)  OutDataTypeStr=fixdt(1,32,0)
  Scope : Scope  NumInputPorts=4
  Output : Outport
  wires:
  Input/1 -> Scope/1, ConvertIn/1
  ConvertIn/1 -> Scope/2, IntSum2/1
  IntSum2/1 -> IntDelay2/1
  IntDelay2/1 -> IntSum3/1, IntSum2/2
  IntSum3/1 -> IntDelay3/1
  IntDelay3/1 -> IntSum1/1, IntSum3/2
  IntSum1/1 -> IntDelay4/1
  IntDelay4/1 -> IntSum1/2, Down Sample/1
  Down Sample/1 -> CombCast6/1
  CombSum3/1 -> CombSum4/1, CombDelay7/1
  CombDelay6/1 -> CombSum3/2
  CombCast6/1 -> Scope/3, CombSum3/1, CombDelay6/1
  CombSum4/1 -> CombSum1/1, CombDelay8/1
  CombDelay7/1 -> CombSum4/2
  CombSum1/1 -> ConvertOut/1
  CombDelay8/1 -> CombSum1/2
  ConvertOut/1 -> Scope/4, Output/1

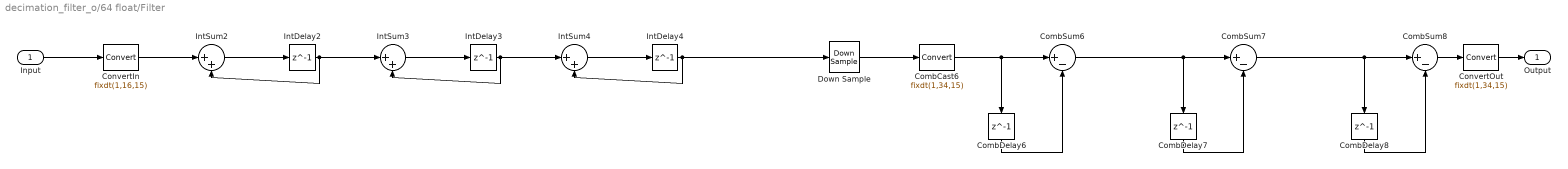
== system decimation_filter_o/64 float/Filter ==
  Input : Inport
  CombCast6 : DataTypeConversion  OutDataTypeStr=fixdt(1,34,15)
  CombDelay6 : Delay  DelayLength=1  InitialCondition=0
  CombDelay7 : Delay  DelayLength=1  InitialCondition=0
  CombDelay8 : Delay  DelayLength=1  InitialCondition=0
  CombSum6 : Sum  Inputs=|+-  AccumDataTypeStr=fixdt(1,34,15)  OutDataTypeStr=fixdt(1,34,15)
  CombSum7 : Sum  Inputs=|+-  AccumDataTypeStr=fixdt(1,34,15)  OutDataTypeStr=fixdt(1,34,15)
  CombSum8 : Sum  Inputs=|+-  AccumDataTypeStr=fixdt(1,34,15)  OutDataTypeStr=fixdt(1,34,15)
  ConvertIn : DataTypeConversion  OutDataTypeStr=fixdt(1,16,15)  RndMeth=Nearest  SaturateOnIntegerOverflow=on
  ConvertOut : DataTypeConversion  OutDataTypeStr=fixdt(1,34,15)
  Down Sample : DownSample  N=64  RateOptions=Allow multirate processing
  IntDelay2 : Delay  DelayLength=1  InitialCondition=0
  IntDelay3 : Delay  DelayLength=1  InitialCondition=0
  IntDelay4 : Delay  DelayLength=1  InitialCondition=0
  IntSum2 : Sum  Inputs=|++  AccumDataTypeStr=fixdt(1,34,15)  OutDataTypeStr=fixdt(1,34,15)
  IntSum3 : Sum  Inputs=|++  AccumDataTypeStr=fixdt(1,34,15)  OutDataTypeStr=fixdt(1,34,15)
  IntSum4 : Sum  Inputs=|++  AccumDataTypeStr=fixdt(1,34,15)  OutDataTypeStr=fixdt(1,34,15)
  Output : Outport
  wires:
  Input/1 -> ConvertIn/1
  ConvertIn/1 -> IntSum2/1
  IntSum2/1 -> IntDelay2/1
  IntDelay2/1 -> IntSum2/2, IntSum3/1
  IntSum3/1 -> IntDelay3/1
  IntDelay3/1 -> IntSum3/2, IntSum4/1
  IntSum4/1 -> IntDelay4/1
  IntDelay4/1 -> IntSum4/2, Down Sample/1
  Down Sample/1 -> CombCast6/1
  CombSum6/1 -> CombSum7/1, CombDelay7/1
  CombDelay6/1 -> CombSum6/2
  CombCast6/1 -> CombSum6/1, CombDelay6/1
  CombSum7/1 -> CombSum8/1, CombDelay8/1
  CombDelay7/1 -> CombSum7/2
  CombSum8/1 -> ConvertOut/1
  CombDelay8/1 -> CombSum8/2
  ConvertOut/1 -> Output/1

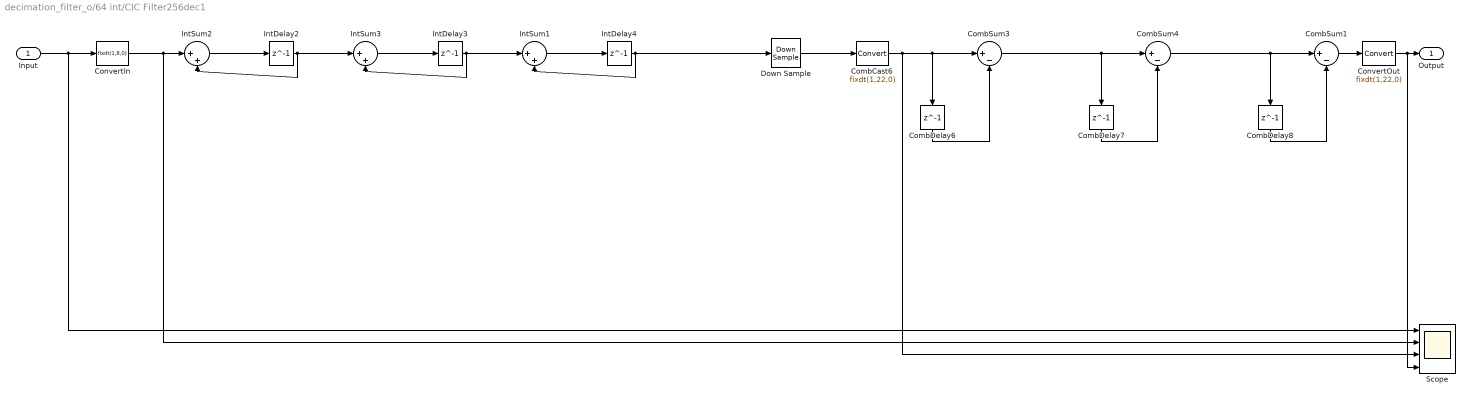
== system decimation_filter_o/64 int/CIC Filter256dec1 ==
  Input : Inport
  CombCast6 : DataTypeConversion  OutDataTypeStr=fixdt(1,22,0)
  CombDelay6 : Delay  DelayLength=1  InitialCondition=0
  CombDelay7 : Delay  DelayLength=1  InitialCondition=0
  CombDelay8 : Delay  DelayLength=1  InitialCondition=0
  CombSum1 : Sum  Inputs=|+-  AccumDataTypeStr=fixdt(1,28,0)  OutDataTypeStr=fixdt(1,28,0)
  CombSum3 : Sum  Inputs=|+-  AccumDataTypeStr=fixdt(1,28,0)  OutDataTypeStr=fixdt(1,28,0)
  CombSum4 : Sum  Inputs=|+-  AccumDataTypeStr=fixdt(1,28,0)  OutDataTypeStr=fixdt(1,28,0)
  ConvertIn : DataTypeConversion  OutDataTypeStr=fixdt(1,8,0)  RndMeth=Nearest  SaturateOnIntegerOverflow=on
  ConvertOut : DataTypeConversion  OutDataTypeStr=fixdt(1,22,0)
  Down Sample : DownSample  N=64  RateOptions=Allow multirate processing
  IntDelay2 : Delay  DelayLength=1  InitialCondition=0
  IntDelay3 : Delay  DelayLength=1  InitialCondition=0
  IntDelay4 : Delay  DelayLength=1  InitialCondition=0
  IntSum1 : Sum  Inputs=|++  AccumDataTypeStr=fixdt(1,30,0)  OutDataTypeStr=fixdt(1,30,0)
  IntSum2 : Sum  Inputs=|++  AccumDataTypeStr=fixdt(1,30,0)  OutDataTypeStr=fixdt(1,30,0)
  IntSum3 : Sum  Inputs=|++  AccumDataTypeStr=fixdt(1,30,0)  OutDataTypeStr=fixdt(1,32,0)
  Scope : Scope  NumInputPorts=4
  Output : Outport
  wires:
  Input/1 -> Scope/1, ConvertIn/1
  ConvertIn/1 -> Scope/2, IntSum2/1
  IntSum2/1 -> IntDelay2/1
  IntDelay2/1 -> IntSum3/1, IntSum2/2
  IntSum3/1 -> IntDelay3/1
  IntDelay3/1 -> IntSum1/1, IntSum3/2
  IntSum1/1 -> IntDelay4/1
  IntDelay4/1 -> IntSum1/2, Down Sample/1
  Down Sample/1 -> CombCast6/1
  CombSum3/1 -> CombSum4/1, CombDelay7/1
  CombDelay6/1 -> CombSum3/2
  CombCast6/1 -> Scope/3, CombSum3/1, CombDelay6/1
  CombSum4/1 -> CombSum1/1, CombDelay8/1
  CombDelay7/1 -> CombSum4/2
  CombSum1/1 -> ConvertOut/1
  CombDelay8/1 -> CombSum1/2
  ConvertOut/1 -> Scope/4, Output/1
